simulink subsystem "OneActuatorAWD"  (R2022b)
settings: Solver=VariableStepAuto  StartTime=0.0  StopTime=10.0  RelTol=1e-3
settings Model: Creator=The MathWorks, Inc.  LastModifiedBy=The MathWorks, Inc.

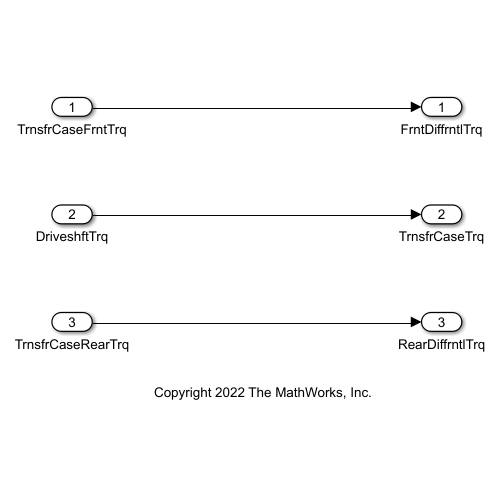
[thumbnail: Simulink's stored preview of the top-level diagram]
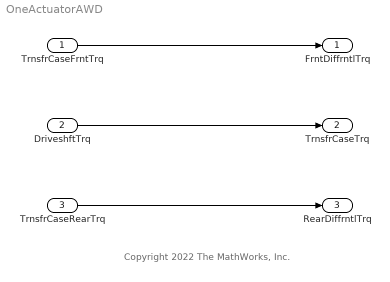
== system OneActuatorAWD ==
  note: Copyright 2022 The MathWorks, Inc.
  TrnsfrCaseFrntTrq : Inport
  DriveshftTrq : Inport  Port=2
  TrnsfrCaseRearTrq : Inport  Port=3
  FrntDiffrntlTrq : Outport
  TrnsfrCaseTrq : Outport  Port=2
  RearDiffrntlTrq : Outport  Port=3
  wires:
  TrnsfrCaseRearTrq/1 -> RearDiffrntlTrq/1
  TrnsfrCaseFrntTrq/1 -> FrntDiffrntlTrq/1
  DriveshftTrq/1 -> TrnsfrCaseTrq/1
